simulink model "Tutorial3_UART"  (R2020a)
settings: Solver=FixedStepAuto  StartTime=0.0  StopTime=10.0  FixedStep=1e-3  RelTol=1e-3  EnableMultiTasking=on
libraries: frdmk64flib x5, etargetslib x2
settings Model: ExtModeTrigDuration=5  Creator=haque  LastModifiedBy=haque
settings OptimizationCC: EnhancedBackFolding=on  PassReuseOutputArgsAs=Individual arguments  ZeroExternalMemoryAtStartup=off  ZeroInternalMemoryAtStartup=off  MaxStackSize=64  OptimizeBlockOrder=speed  DifferentSizesBufferReuse=on  OptimizationCustomize=off  EfficientTunableParamExpr=on
settings DebuggingCC: ParameterTunabilityLossMsg=error
settings HardwareCC: ProdBitPerPointer=32  ProdBitPerSizeT=32  ProdBitPerPtrDiffT=32  ProdLargestAtomicInteger=Long  ProdLargestAtomicFloat=Double  ProdWordSize=32  ProdHWDeviceType=ARM Compatible->ARM Cortex
settings SFSimCC: MATLABDynamicMemAlloc=off
settings RTWCC: SystemTargetFile=ert.tlc  HardwareBoard=NXP FRDM-K64F  TemplateMakefile=ert_default_tmf  Toolchain=GNU Tools for ARM Embedded Processors
settings CodeAppCC: ForceParamTrailComments=on  IgnoreCustomStorageClasses=off  OperatorAnnotations=on  SimulinkDataObjDesc=on  SFDataObjDesc=on  InsertBlockDesc=on

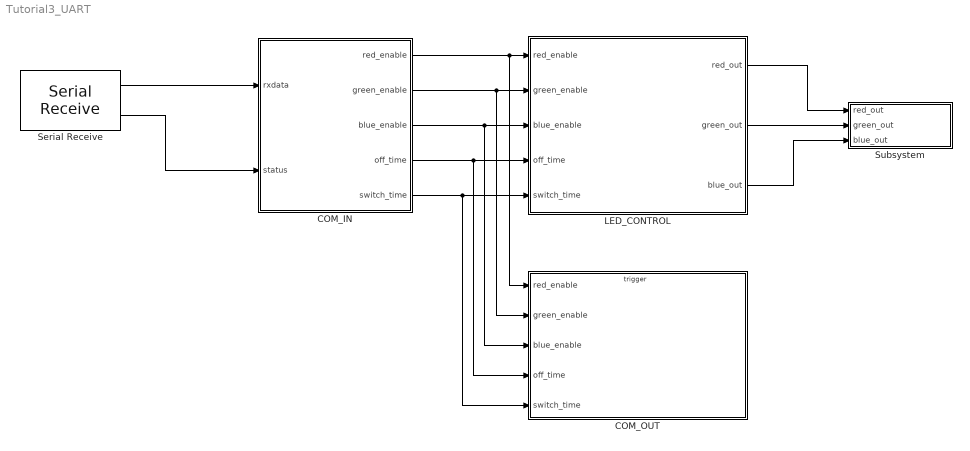
== system Tutorial3_UART ==
  COM_IN : Stateflow chart  TreatAsAtomicUnit=on
  COM_OUT : Subsystem
  LED_CONTROL : Stateflow chart  TreatAsAtomicUnit=on
  Serial Receive : frdmk64flib/Serial Receive  SCIModule=0  Baudrate=uint32(9600)  Parity=None  StopBits=1  HardwareFlowControl=None  ByteOrder=LittleEndian  DataType=uint8  DataLength=11  BlockingMode=off  OutputStatus=on  SampleTime=-1
  Subsystem : Subsystem
  wires:
  Serial Receive/1 -> COM_IN/1(rxdata)
  Serial Receive/2 -> COM_IN/2(status)
  COM_IN/1(red_enable) -> COM_OUT/1(red_enable), LED_CONTROL/1(red_enable)
  COM_IN/2(green_enable) -> COM_OUT/2(green_enable), LED_CONTROL/2(green_enable)
  COM_IN/3(blue_enable) -> COM_OUT/3(blue_enable), LED_CONTROL/3(blue_enable)
  COM_IN/4(off_time) -> COM_OUT/4(off_time), LED_CONTROL/4(off_time)
  COM_IN/5(switch_time) -> COM_OUT/5(switch_time), LED_CONTROL/5(switch_time)
  LED_CONTROL/1(red_out) -> Subsystem/1(red_out)
  LED_CONTROL/2(green_out) -> Subsystem/2(green_out)
  LED_CONTROL/3(blue_out) -> Subsystem/3(blue_out)

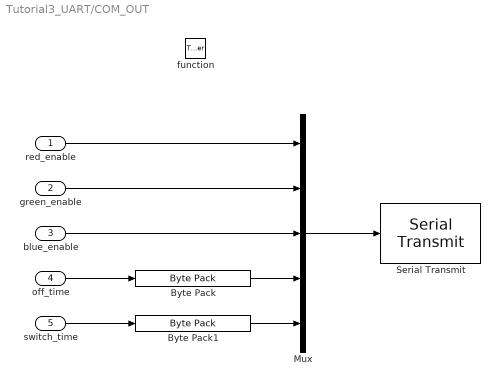
== system Tutorial3_UART/COM_OUT ==
  red_enable : Inport
  green_enable : Inport  Port=2
  blue_enable : Inport  Port=3
  off_time : Inport  Port=4
  switch_time : Inport  Port=5
  function : TriggerPort  TriggerType=function-call  VariantControl=Variant
  Byte Pack : etargetslib/Byte Pack  datatypes={'double'}  byteAlign=1
  Byte Pack1 : etargetslib/Byte Pack  datatypes={'double'}  byteAlign=1
  Mux : Mux  Inputs=5
  Serial Transmit : frdmk64flib/Serial Transmit  SCIModule=0  Baudrate=uint32(9600)  Parity=None  StopBits=1  HardwareFlowControl=None  ByteOrder=LittleEndian  BlockingMode=on  OutputStatus=off
  wires:
  off_time/1 -> Byte Pack/1
  switch_time/1 -> Byte Pack1/1
  red_enable/1 -> Mux/1
  green_enable/1 -> Mux/2
  blue_enable/1 -> Mux/3
  Byte Pack/1 -> Mux/4
  Byte Pack1/1 -> Mux/5
  Mux/1 -> Serial Transmit/1

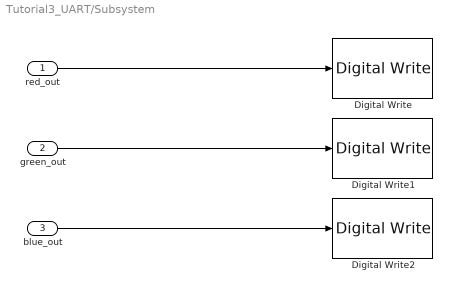
== system Tutorial3_UART/Subsystem ==
  red_out : Inport
  green_out : Inport  Port=2
  blue_out : Inport  Port=3
  Digital Write : frdmk64flib/Digital Write  Whichpin=RED_LED
  Digital Write1 : frdmk64flib/Digital Write  Whichpin=GREEN_LED
  Digital Write2 : frdmk64flib/Digital Write  Whichpin=BLUE_LED
  wires:
  red_out/1 -> Digital Write/1
  green_out/1 -> Digital Write1/1
  blue_out/1 -> Digital Write2/1

== stateflow chart Tutorial3_UART/LED_CONTROL ==
  state OFF
    entry:
    red_out=0;
    green_out=0;
    blue_out=0;
  state RED_ON
    entry:
    red_out=1;
    green_out=0;
    blue_out=0;
  state BLUE_ON
    entry:
    red_out=0;
    green_out=0;
    blue_out=1;
  state GREEN_ON
    entry:
    red_out=0;
    green_out=1;
    blue_out=0;
  (default) -> OFF
  OFF -> (junction 15) : [after(off_time, sec)]
  (junction 15) -> RED_ON [order 1] : [red_enable==1]
  (junction 15) -> (junction 16) [order 2]
  (junction 14) -> OFF
  RED_ON -> (junction 16) : [after(switch_time, msec)]
  (junction 17) -> (junction 14) [order 2]
  (junction 16) -> (junction 17) [order 2]
  BLUE_ON -> (junction 14) : [[after(switch_time, msec)]]
  (junction 16) -> GREEN_ON [order 1] : [green_enable==1]
  (junction 17) -> BLUE_ON [order 1] : [blue_enable==1]
  GREEN_ON -> (junction 17) : [after(switch_time, msec)]
  data: red_enable input; green_enable input; blue_enable input; off_time input; switch_time input; red_out output; green_out output; blue_out output

== stateflow chart Tutorial3_UART/COM_IN ==
  settings: executeAtInitialization=1
  state SET_PARAM
    entry:
    red_enable=rxdata(3);
    green_enable=rxdata(4);
    blue_enable=rxdata(5);
    off_time=typecast(rxdata(6:9), 'single');
    switch_time=typecast(rxdata(10:11), 'uint16');
  state INITIAL
    % Set the initial values of parameters
    entry:
    red_enable=1;
    green_enable=1;
    blue_enable=0;
    off_time=0.5; % in s
    switch_time=200; %in ms
  state STANDBY
    % waiting for COM
  state ECHO_PARAM
    entry:
    send_params();
  SET_PARAM -> STANDBY
  (default) -> INITIAL
  (junction 16) -> SET_PARAM [order 1] : [rxdata(2) == hex2dec('55')]
  (junction 15) -> STANDBY [order 2]
  INITIAL -> STANDBY
  STANDBY -> (junction 15) : [status == 0]
  (junction 15) -> (junction 16) [order 1] : [rxdata(1) == hex2dec('16')]
  (junction 16) -> ECHO_PARAM [order 2] : [rxdata(2) == hex2dec('22')]
  data: rxdata input; status input; red_enable output; green_enable output; blue_enable output; off_time output; switch_time output
